simulink model "Erreurv"  (R2017b)
settings: Solver=FixedStepDiscrete  StartTime=0.0  StopTime=2  FixedStep=Te  RelTol=1e-3  EnableMultiTasking=on
undefined symbols (not defined in the file): DKp1, DP, NKp1, NP, Te
libraries: simulink x1
settings Model: Creator=Avisse  LastModifiedBy=lencs
settings DataIOCC: LimitDataPoints=on  SaveFormat=Array
settings OptimizationCC: LifeSpan=inf
settings DebuggingCC: SolverPrmCheckMsg=warning  SFUnexpectedBacktrackingDiag=warning  SFNoUnconditionalDefaultTransitionDiag=warning  SFExecutionAtInitializationDiag=none
settings HardwareCC: ProdBitPerPointer=32  ProdBitPerSizeT=32  ProdBitPerPtrDiffT=32  ProdLargestAtomicFloat=None  ProdIntDivRoundTo=Undefined  ProdEndianess=Unspecified  ProdWordSize=32  ProdHWDeviceType=32-bit Generic
settings ModelReferenceCC: PropagateSignalLabelsOutOfModel=off
settings CodeAppCC: StateflowObjectComments=on
settings GRTTargetCC: TargetLangStandard=C89/C90 (ANSI)  GeneratePreprocessorConditionals=Disable all
settings ConfigComp: CovMetricSettings=dw  CovHtmlReporting=on  CovSaveCumulativeToWorkspaceVar=on  CovSaveSingleToWorkspaceVar=on  CovExternalEMLEnable=off  CovSFcnEnable=off

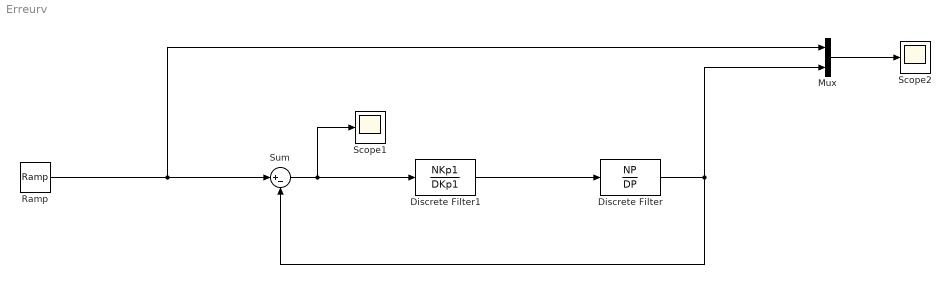
== system Erreurv ==
  Discrete Filter : DiscreteFilter  Numerator=NP  Denominator=DP  SampleTime=Te
  Discrete Filter1 : DiscreteFilter  Numerator=NKp1  Denominator=DKp1  SampleTime=Te
  Mux : Mux  Inputs=2
  Ramp : simulink/Sources/Ramp  slope=1  start=0  X0=0
  Scope1 : Scope
  Scope2 : Scope
  Sum : Sum  Inputs=|+-
  wires:
  Mux/1 -> Scope2/1
  Ramp/1 -> Mux/1, Sum/1
  Discrete Filter/1 -> Sum/2, Mux/2
  Sum/1 -> Scope1/1, Discrete Filter1/1
  Discrete Filter1/1 -> Discrete Filter/1
